simulink model "FINAL_MLC_IPC_0_r2018a"  (Simulink 9.1)
settings: Solver=ode4  StartTime=0.0  StopTime=Parameter.Time.TMax  FixedStep=Parameter.Time.dt  RelTol=1e-3  EnableMultiTasking=on
undefined symbols (not defined in the file or in its folder): OutList, Parameter, strmatch, x2_t0
libraries: simulink x13
(part 2 of 2)

== matlab function MLC_IPC/pitch_ctrl_1/direct_signal ==
  data: u input double; y output double
function y = fcn(u)
y = 0;

== matlab function MLC_IPC/pitch_ctrl_1/integral_signal ==
  data: u input double; y output double
function y = fcn(u)
y = 0;

== matlab function MLC_IPC/pitch_ctrl_2/direct_signal ==
  data: u input double; y output double
function y = fcn(u)
y = 0;

== matlab function MLC_IPC/pitch_ctrl_2/integral_signal ==
  data: u input double; y output double
function y = fcn(u)
y = 0;

== matlab function MLC_IPC/pitch_ctrl_3/direct_signal ==
  data: u input double; y output double
function y = fcn(u)
y = 0;

== matlab function MLC_IPC/pitch_ctrl_3/integral_signal ==
  data: u input double; y output double
function y = fcn(u)
y = 0;
